simulink model "of_guidance"  (R2017b)
settings: Solver=FixedStepDiscrete  StartTime=0.0  StopTime=inf  FixedStep=0.01  RelTol=1e-3
undefined symbols (not defined in the file): Data, Data_SL_Info, DiscIntNeverNeededParam, Y_Velocity
libraries: robotlib x6, dspstat3 x5, simulink x3
settings Model: Creator=a  LastModifiedBy=a
settings OptimizationCC: PassReuseOutputArgsAs=Individual arguments  MaxStackSize=64
settings DebuggingCC: ParameterTunabilityLossMsg=error
settings HardwareCC: ProdBitPerPointer=32  ProdBitPerSizeT=32  ProdBitPerPtrDiffT=32  ProdLargestAtomicFloat=None  ProdIntDivRoundTo=Undefined  ProdEndianess=Unspecified  ProdWordSize=32  ProdHWDeviceType=Generic->Unspecified (assume 32-bit Generic)
settings SFSimCC: MATLABDynamicMemAlloc=off
settings RTWCC: SystemTargetFile=ert.tlc  HardwareBoard=Robot Operating System (ROS)  TemplateMakefile=ert_default_tmf  GenerateReport=on  Toolchain=Catkin  IncludeHyperlinkInReport=on  LaunchReport=on  TargetLang=C++  GenerateTraceInfo=on  GenerateTraceReport=on  GenerateTraceReportSl=on  GenerateTraceReportSf=on  GenerateTraceReportEml=on
settings CodeAppCC: ForceParamTrailComments=on  IgnoreCustomStorageClasses=off  OperatorAnnotations=on  SimulinkDataObjDesc=on  SFDataObjDesc=on  InsertBlockDesc=on

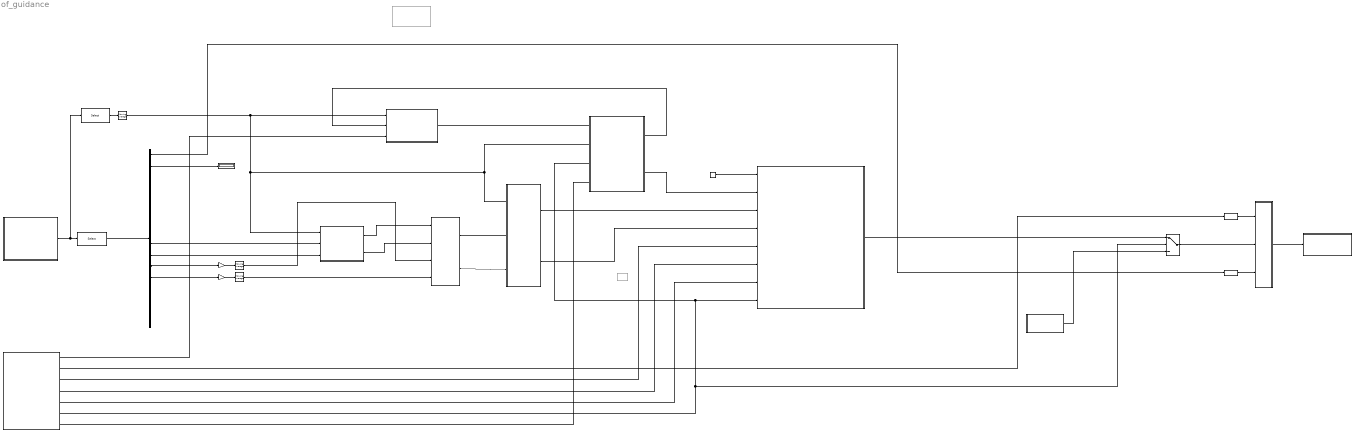
== system of_guidance ==
  Data Type Conversion3 : DataTypeConversion  OutDataTypeStr=single
  Data Type Conversion4 : DataTypeConversion  OutDataTypeStr=single
  Demux : Demux  Outputs=16
  P Moving Average : dspstat3/Moving Average  Method=Sliding window  SpecifyWindowLength=on  WindowLength=35  ForgettingFactor=0.9  SimulateUsing=Code generation
  Q Moving Average : dspstat3/Moving Average  Method=Sliding window  SpecifyWindowLength=on  WindowLength=35  ForgettingFactor=0.9  SimulateUsing=Code generation
  Selector : Selector  InputPortWidth=26  IndexOptions=Index vector (dialog)  Indices=[17:26 4 5 6 11 12 13]  OutputSizes=1
  Selector1 : Selector  InputPortWidth=26  IndexOptions=Index vector (dialog)  Indices=[7]  OutputSizes=1
  Sonar Moving Average : dspstat3/Moving Average  Method=Sliding window  SpecifyWindowLength=on  WindowLength=5  ForgettingFactor=0.9  SimulateUsing=Code generation
  Subsystem2 : Subsystem
  Subsystem5 : Subsystem
  Switch : Switch  Criteria=u2 > Threshold
  check_arm_status : Subsystem
  command_input : Subsystem
  command_output : Subsystem
  compensate_angular_velocity_effect_on_of : Subsystem
  "data_input " : Subsystem
  manual_control : Subsystem  mask{throttle=0.0, roll=0, pitch=0, yaw=0, mode=0}
  manual_throttle : Subsystem  Commented=on  mask{th=90}
  mode : Constant  Value=2
  p gain : Gain  Gain=3.1415 / 180.0
  pixel_per_sec_to_m_per_sec : Subsystem
  q gain : Gain  Gain=3.1415 / 180.0
  radio_command_frame_rate : Display
  throttle_handler_climb_mode : Subsystem
  velocity_control : Subsystem
  vy_setpoint1 : Constant  Commented=on  Value=Y_Velocity
  wires:
  command_input/5(vx_des) -> velocity_control/7(vx_setpoint)
  Selector/1 -> Demux/1
  pixel_per_sec_to_m_per_sec/2(vy(m/s)) -> compensate_angular_velocity_effect_on_of/2(vy)
  Demux/2 -> radio_command_frame_rate/1
  Switch/1 -> check_arm_status/2(command)
  command_input/6(take_off) -> Switch/2, velocity_control/8(Integrator_reset), throttle_handler_climb_mode/3(integrator_reset)
  Subsystem2/1(throttle_command) -> throttle_handler_climb_mode/1(desired_throttle)
  command_input/3(yaw_rate_des) -> velocity_control/5(yaw_des_rate)
  throttle_handler_climb_mode/1(z_controller_integrator_reset) -> Subsystem2/2(integrator_reset)
  command_input/1(z_des) -> Subsystem2/3(z_desired)
  command_input/4(vy_des) -> velocity_control/6(vy_setpoint)
  command_input/7(landing) -> throttle_handler_climb_mode/4(landing)
  Demux/12 -> q gain/1
  velocity_control/1(radio_command) -> Switch/1
  Subsystem5/2(vy_out) -> velocity_control/4(vy)
  Demux/11 -> p gain/1
  Demux/10 -> pixel_per_sec_to_m_per_sec/3(vy(pix/sec))
  "data_input "/1(data) -> Selector/1, Selector1/1
  command_input/2(arm_status) -> Data Type Conversion4/1
  Demux/9 -> pixel_per_sec_to_m_per_sec/2(vx(pix/sec))
  compensate_angular_velocity_effect_on_of/1(corrected_vx) -> Subsystem5/2(vx)
  p gain/1 -> P Moving Average/1
  q gain/1 -> Q Moving Average/1
  pixel_per_sec_to_m_per_sec/1(vx(m/s)) -> compensate_angular_velocity_effect_on_of/1(vx)
  P Moving Average/1 -> compensate_angular_velocity_effect_on_of/3(p)
  Data Type Conversion4/1 -> check_arm_status/1(arm)
  manual_control/1(commands) -> Switch/3
  Subsystem5/1(vx_out) -> velocity_control/3(vx)
  Data Type Conversion3/1 -> check_arm_status/3(motors_on)
  check_arm_status/1(Out) -> command_output/1(command)
  Sonar Moving Average/1 -> pixel_per_sec_to_m_per_sec/1(height), Subsystem5/1(height), throttle_handler_climb_mode/2(height), Subsystem2/1(measured_height)
  mode/1 -> velocity_control/1(mode)
  throttle_handler_climb_mode/2(throttle) -> velocity_control/2(throttle)
  Demux/1 -> Data Type Conversion3/1
  Selector1/1 -> Sonar Moving Average/1
  compensate_angular_velocity_effect_on_of/2(corrected_vy) -> Subsystem5/3(vy)
  Q Moving Average/1 -> compensate_angular_velocity_effect_on_of/4(q)

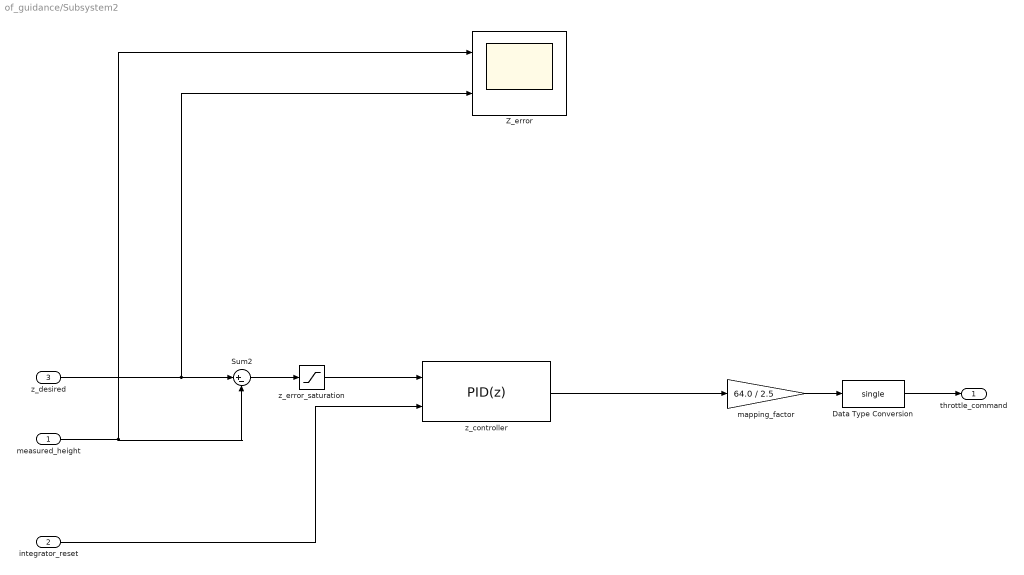
== system of_guidance/Subsystem2 ==
  measured_height : Inport
  integrator_reset : Inport  Port=2
  z_desired : Inport  Port=3
  Data Type Conversion : DataTypeConversion  OutDataTypeStr=single
  Sum2 : Sum  Inputs=|+-
  Z_error : Scope  NumInputPorts=2
  mapping_factor : Gain  Gain=64.0 / 2.5
  z_controller : simulink/Continuous/PID Controller  Controller=PID  TimeDomain=Discrete-time  SampleTime=-1  IntegratorMethod=Forward Euler  FilterMethod=Forward Euler  Form=Parallel  UseFilter=on  ControllerParametersSource=internal  P=1.5  I=0.3  D=0.2  N=100  InitialConditionSource=internal  InitialConditionForIntegrator=0  InitialConditionForFilter=0  ExternalReset=rising  LimitOutput=on  UpperSaturationLimit=1.0  LowerSaturationLimit=-1.0  LinearizeAsGain=off  AntiWindupMode=none  Kb=1  TrackingMode=off  Kt=1  PParamMin=[]  PParamMax=[]  IParamMin=[]  IParamMax=[]  DParamMin=[]  DParamMax=[]  NParamMin=[]  NParamMax=[]  KbParamMin=[]  KbParamMax=[]  KtParamMin=[]  KtParamMax=[]  POutMin=[]  POutMax=[]  IOutMin=[]  IOutMax=[]  DOutMin=[]  DOutMax=[]  NOutMin=[]  NOutMax=[]  KbOutMin=[]  KbOutMax=[]  KtOutMin=[]  KtOutMax=[]  IntegratorOutMin=[]  IntegratorOutMax=[]  FilterOutMin=[]  FilterOutMax=[]  SumOutMin=[]  SumOutMax=[]  SumI1OutMin=[]  SumI1OutMax=[]  SumI2OutMin=[]  SumI2OutMax=[]  SumI3OutMin=[]  SumI3OutMax=[]  SumDOutMin=[]  SumDOutMax=[]  SaturationOutMin=[]  SaturationOutMax=[]  IntegratorContinuousStateAttributes=''  IntegratorStateMustResolveToSignalObject=off  IntegratorRTWStateStorageClass=Auto  FilterContinuousStateAttributes=''  FilterStateMustResolveToSignalObject=off  FilterRTWStateStorageClass=Auto  DifferentiatorICPrevScaledInput=0  DifferentiatorOutMin=[]  DifferentiatorOutMax=[]  InitialConditionSetting=State (most efficient)  FilterDiffOutCoefMin=[]  FilterDiffOutCoefMax=[]  SumDenOutMin=[]  SumDenOutMax=[]  SumNumOutMin=[]  SumNumOutMax=[]  ReciprocalOutMin=[]  ReciprocalOutMax=[]  DivideOutMin=[]  DivideOutMax=[]  TunerSelectOption=Transfer Function Based (PID Tuner App)
  z_error_saturation : Saturate  UpperLimit=1  LowerLimit=-1
  throttle_command : Outport
  wires:
  integrator_reset/1 -> z_controller/2
  mapping_factor/1 -> Data Type Conversion/1
  measured_height/1 -> Sum2/2, Z_error/1
  z_desired/1 -> Z_error/2, Sum2/1
  Sum2/1 -> z_error_saturation/1
  z_error_saturation/1 -> z_controller/1
  z_controller/1 -> mapping_factor/1
  Data Type Conversion/1 -> throttle_command/1

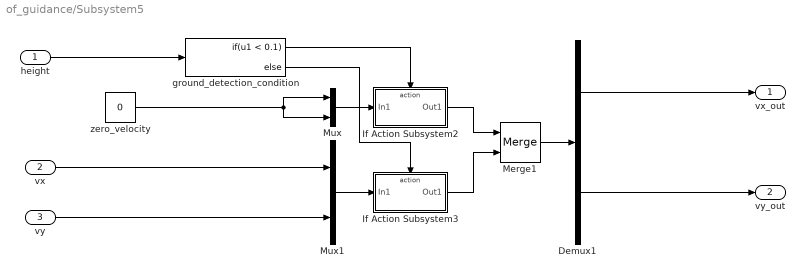
== system of_guidance/Subsystem5 ==
  height : Inport
  vx : Inport  Port=2
  vy : Inport  Port=3
  Demux1 : Demux  Outputs=2
  If Action Subsystem2 : Subsystem  TreatAsAtomicUnit=on
  If Action Subsystem3 : Subsystem  TreatAsAtomicUnit=on
  Merge1 : Merge
  Mux : Mux  Inputs=2
  Mux1 : Mux  Inputs=2
  ground_detection_condition : If  IfExpression=u1 < 0.1
  zero_velocity : Constant  Value=0
  vx_out : Outport
  vy_out : Outport  Port=2
  wires:
  vy/1 -> Mux1/2
  vx/1 -> Mux1/1
  height/1 -> ground_detection_condition/1
  Demux1/1 -> vx_out/1
  zero_velocity/1 -> Mux/2, Mux/1
  Demux1/2 -> vy_out/1
  ground_detection_condition/1 -> If Action Subsystem2/Action
  If Action Subsystem3/1(Out1) -> Merge1/2
  Merge1/1 -> Demux1/1
  Mux1/1 -> If Action Subsystem3/1(In1)
  ground_detection_condition/2 -> If Action Subsystem3/Action
  If Action Subsystem2/1(Out1) -> Merge1/1
  Mux/1 -> If Action Subsystem2/1(In1)

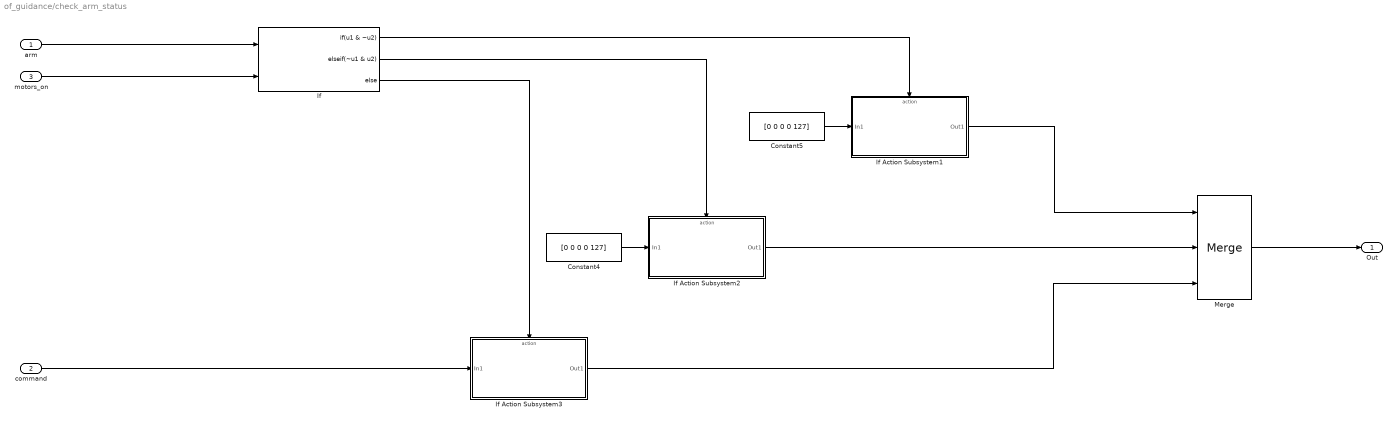
== system of_guidance/check_arm_status ==
  arm : Inport
  command : Inport  Port=2
  motors_on : Inport  Port=3
  Constant4 : Constant  Value=[0 0 0 0 127]
  Constant5 : Constant  Value=[0 0 0 0 127]
  If : If  NumInputs=2  IfExpression=u1 & ~u2  ElseIfExpressions=~u1 & u2
  If Action Subsystem1 : Subsystem  TreatAsAtomicUnit=on
  If Action Subsystem2 : Subsystem  TreatAsAtomicUnit=on
  If Action Subsystem3 : Subsystem  TreatAsAtomicUnit=on
  Merge : Merge  Inputs=3
  Out : Outport
  wires:
  If/1 -> If Action Subsystem1/Action
  Constant4/1 -> If Action Subsystem2/1(In1)
  If/3 -> If Action Subsystem3/Action
  Constant5/1 -> If Action Subsystem1/1(In1)
  If/2 -> If Action Subsystem2/Action
  If Action Subsystem2/1(Out1) -> Merge/2
  motors_on/1 -> If/2
  command/1 -> If Action Subsystem3/1(In1)
  If Action Subsystem1/1(Out1) -> Merge/1
  If Action Subsystem3/1(Out1) -> Merge/3
  arm/1 -> If/1
  Merge/1 -> Out/1

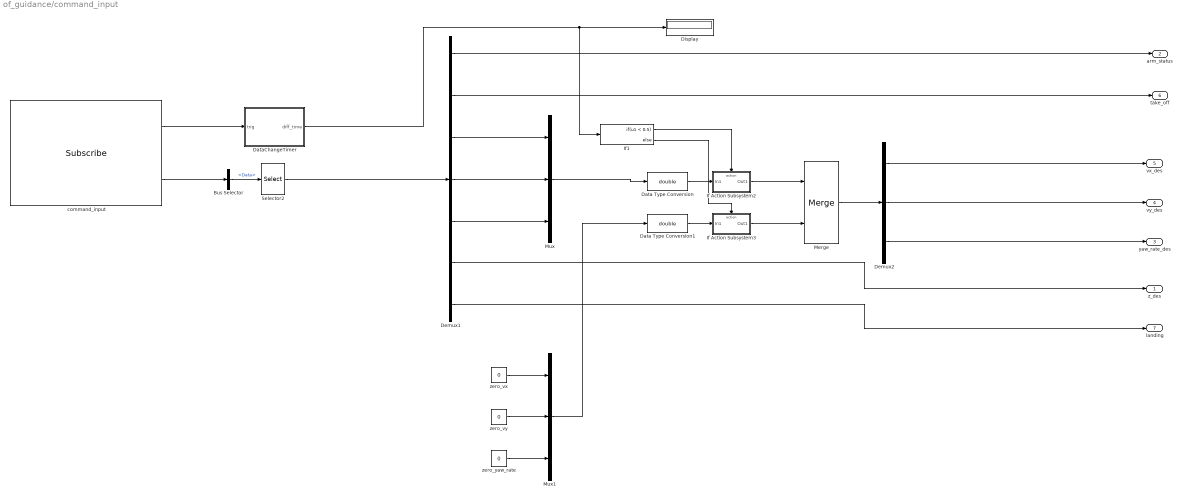
== system of_guidance/command_input ==
  Bus Selector : BusSelector  OutputSignals=Data
  Data Type Conversion : DataTypeConversion  OutDataTypeStr=double
  Data Type Conversion1 : DataTypeConversion  OutDataTypeStr=double
  DataChangeTimer : Subsystem
  Demux1 : Demux  Outputs=7
  Demux2 : Demux  Outputs=3
  Display : Display
  If Action Subsystem2 : Subsystem  TreatAsAtomicUnit=on
  If Action Subsystem3 : Subsystem  TreatAsAtomicUnit=on
  If1 : If  IfExpression=u1 < 0.5
  Merge : Merge
  Mux : Mux  Inputs=3
  Mux1 : Mux  Inputs=3
  Selector2 : Selector  InputPortWidth=128  IndexOptions=Index vector (dialog)  Indices=[1 2 3 4 5 6 7]  OutputSizes=1
  command_input : robotlib/Subscribe  SourceLibraryInfo=This block requires Robotics System Toolbox  topicSource=Specify your own  topic=/quadrotor_1/road_following_cmd  messageType=std_msgs/Float32MultiArray  sampleTime=-1  messageQueueLength=1
      settings: SourceProductBaseCode=RO
  zero_vx : Constant  Value=0
  zero_vy : Constant  Value=0
  zero_yaw_rate : Constant  Value=0
  z_des : Outport
  arm_status : Outport  Port=2
  yaw_rate_des : Outport  Port=3
  vy_des : Outport  Port=4
  vx_des : Outport  Port=5
  take_off : Outport  Port=6
  landing : Outport  Port=7
  wires:
  DataChangeTimer/1(diff_time) -> If1/1, Display/1
  If1/2 -> If Action Subsystem3/Action
  Demux1/5 -> Mux/3
  Demux1/1 -> arm_status/1
  Demux2/1 -> vx_des/1
  If1/1 -> If Action Subsystem2/Action
  Demux1/4 -> Mux/2
  command_input/1 -> DataChangeTimer/1(trig)
  Mux/1 -> Data Type Conversion/1
  command_input/2 -> Bus Selector/1
  Bus Selector/1 -> Selector2/1  "<Data>"
  Demux1/2 -> take_off/1
  Demux2/2 -> vy_des/1
  Demux1/6 -> z_des/1
  Demux2/3 -> yaw_rate_des/1
  Selector2/1 -> Demux1/1
  zero_yaw_rate/1 -> Mux1/3
  zero_vx/1 -> Mux1/1
  Mux1/1 -> Data Type Conversion1/1
  zero_vy/1 -> Mux1/2
  Demux1/3 -> Mux/1
  Merge/1 -> Demux2/1
  Demux1/7 -> landing/1
  If Action Subsystem2/1(Out1) -> Merge/1
  If Action Subsystem3/1(Out1) -> Merge/2
  Data Type Conversion/1 -> If Action Subsystem2/1(In1)
  Data Type Conversion1/1 -> If Action Subsystem3/1(In1)

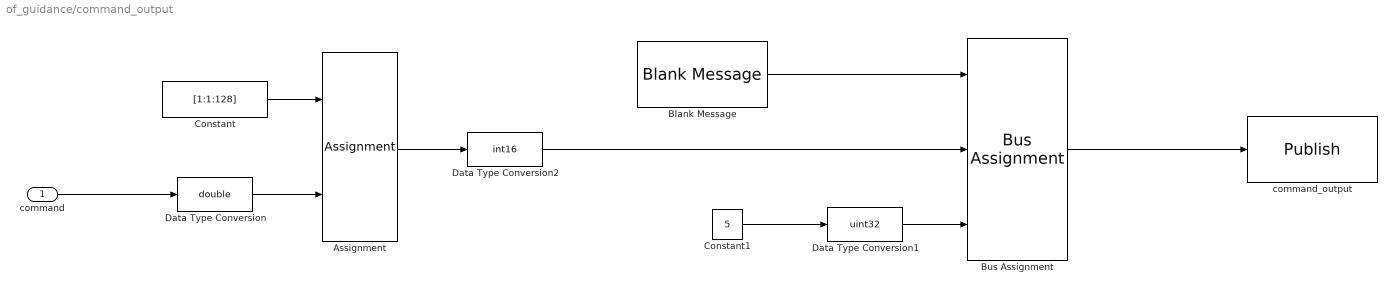
== system of_guidance/command_output ==
  command : Inport
  Assignment : Assignment  DiagnosticForDimensions=Warning  IndexOptions=Index vector (dialog)  Indices=[1 2 3 4 5]  OutputSizes=1
  Blank Message : robotlib/Blank Message  SourceLibraryInfo=This block requires Robotics System Toolbox  messageType=std_msgs/Int16MultiArray  SampleTime=inf
      settings: SourceProductBaseCode=RO
  Bus Assignment : BusAssignment  AssignedSignals=Data,Data_SL_Info.CurrentLength
  Constant : Constant  Value=[1:1:128]
  Constant1 : Constant  Value=5
  Data Type Conversion : DataTypeConversion  OutDataTypeStr=double
  Data Type Conversion1 : DataTypeConversion  OutDataTypeStr=uint32
  Data Type Conversion2 : DataTypeConversion  OutDataTypeStr=int16
  "command_output " : robotlib/Publish  SourceLibraryInfo=This block requires Robotics System Toolbox  topicSource=Select from ROS network  topic=/quadrotor_1/rpyt_command  messageType=std_msgs/Int16MultiArray  messageQueueLength=1
      settings: SourceProductBaseCode=RO
  wires:
  Constant1/1 -> Data Type Conversion1/1
  Data Type Conversion1/1 -> Bus Assignment/3
  Bus Assignment/1 -> "command_output "/1
  Data Type Conversion2/1 -> Bus Assignment/2
  Assignment/1 -> Data Type Conversion2/1
  Blank Message/1 -> Bus Assignment/1
  Data Type Conversion/1 -> Assignment/2
  command/1 -> Data Type Conversion/1
  Constant/1 -> Assignment/1

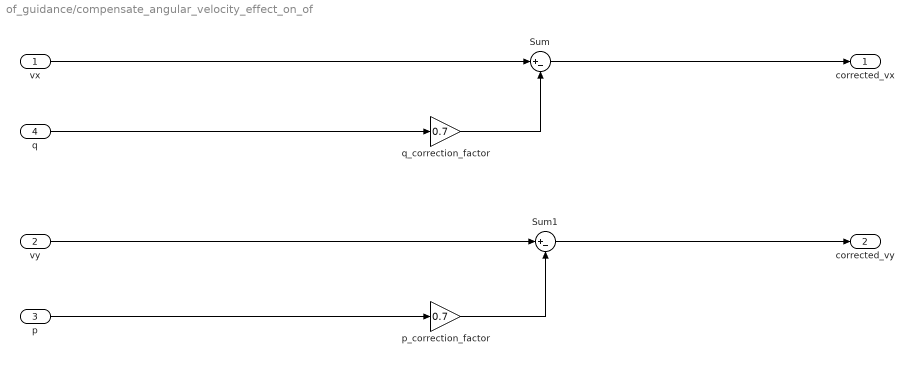
== system of_guidance/compensate_angular_velocity_effect_on_of ==
  vx : Inport
  vy : Inport  Port=2
  p : Inport  Port=3
  q : Inport  Port=4
  Sum : Sum  Inputs=|+-
  Sum1 : Sum  Inputs=|+-
  p_correction_factor : Gain  Gain=0.7
  q_correction_factor : Gain  Gain=0.7
  corrected_vx : Outport
  corrected_vy : Outport  Port=2
  wires:
  vx/1 -> Sum/1
  vy/1 -> Sum1/1
  q/1 -> q_correction_factor/1
  p/1 -> p_correction_factor/1
  Sum1/1 -> corrected_vy/1
  Sum/1 -> corrected_vx/1
  p_correction_factor/1 -> Sum1/2
  q_correction_factor/1 -> Sum/2

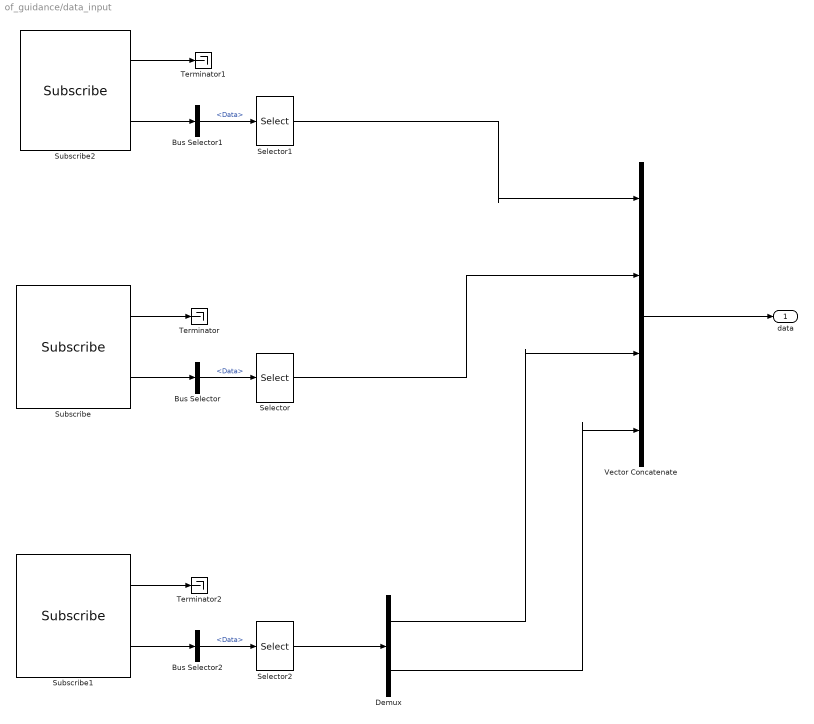
== system of_guidance/data_input  ==
  Bus Selector : BusSelector  OutputSignals=Data
  Bus Selector1 : BusSelector  OutputSignals=Data
  Bus Selector2 : BusSelector  OutputSignals=Data
  Demux : Demux  Outputs=2
  Selector : Selector  InputPortWidth=128  IndexOptions=Index vector (dialog)  Indices=[1 2 3 4 5 6]  OutputSizes=1
  Selector1 : Selector  InputPortWidth=128  IndexOptions=Index vector (dialog)  Indices=[1 2 3 4 5 6 7 8 9 10 11 12 13 14 15 16 17 18]  OutputSizes=1
  Selector2 : Selector  InputPortWidth=128  IndexOptions=Index vector (dialog)  Indices=[1 2]  OutputSizes=1
  Subscribe : robotlib/Subscribe  SourceLibraryInfo=This block requires Robotics System Toolbox  topicSource=Select from ROS network  topic=/quadrotor_1/nav  messageType=std_msgs/Float32MultiArray  sampleTime=-1  messageQueueLength=1
      settings: SourceProductBaseCode=RO
  Subscribe1 : robotlib/Subscribe  SourceLibraryInfo=This block requires Robotics System Toolbox  topicSource=Select from ROS network  topic=/quadrotor_1/optical_flow  messageType=std_msgs/Float32MultiArray  sampleTime=-1  messageQueueLength=1
      settings: SourceProductBaseCode=RO
  Subscribe2 : robotlib/Subscribe  SourceLibraryInfo=This block requires Robotics System Toolbox  topicSource=Select from ROS network  topic=/quadrotor_1/sensor_data  messageType=std_msgs/Float32MultiArray  sampleTime=-1  messageQueueLength=1
      settings: SourceProductBaseCode=RO
  Terminator : Terminator
  Terminator1 : Terminator
  Terminator2 : Terminator
  Vector Concatenate : Concatenate  NumInputs=4
  data : Outport
  wires:
  Subscribe/1 -> Terminator/1
  Selector/1 -> Vector Concatenate/2
  Subscribe2/1 -> Terminator1/1
  Subscribe2/2 -> Bus Selector1/1
  Subscribe/2 -> Bus Selector/1
  Bus Selector/1 -> Selector/1  "<Data>"
  Bus Selector1/1 -> Selector1/1  "<Data>"
  Selector1/1 -> Vector Concatenate/1
  Vector Concatenate/1 -> data/1
  Subscribe1/2 -> Bus Selector2/1
  Subscribe1/1 -> Terminator2/1
  Bus Selector2/1 -> Selector2/1  "<Data>"
  Selector2/1 -> Demux/1
  Demux/1 -> Vector Concatenate/3
  Demux/2 -> Vector Concatenate/4

== system of_guidance/manual_control ==
  Constant : Constant  Value=[mode throttle roll pitch yaw]
  commands : Outport
  wires:
  Constant/1 -> commands/1

== system of_guidance/manual_throttle ==
  mode1 : Constant  Value=th
  Out1 : Outport
  wires:
  mode1/1 -> Out1/1

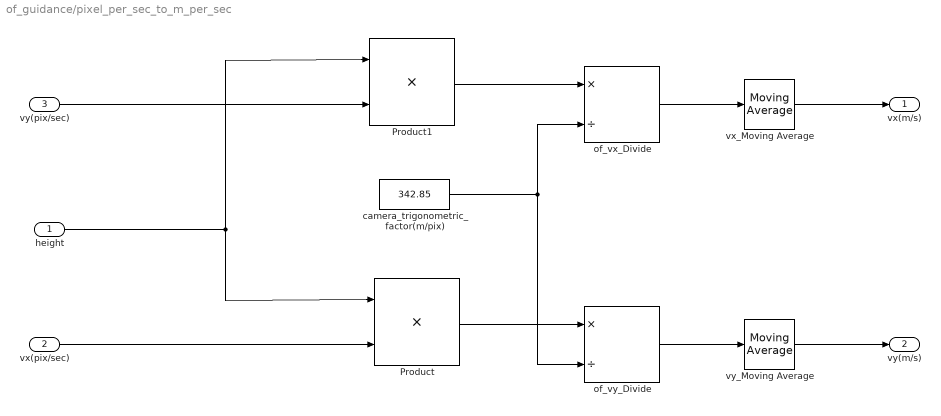
== system of_guidance/pixel_per_sec_to_m_per_sec ==
  height : Inport
  vx(pix/sec) : Inport  Port=2
  vy(pix/sec) : Inport  Port=3
  Product : Product
  Product1 : Product
  camera_trigonometric_factor(m/pix) : Constant  Value=342.85
  of_vx_Divide : Product  Inputs=*/
  of_vy_Divide : Product  Inputs=*/
  vx_Moving Average : dspstat3/Moving Average  Method=Sliding window  SpecifyWindowLength=on  WindowLength=35  ForgettingFactor=0.9  SimulateUsing=Code generation
  vy_Moving Average : dspstat3/Moving Average  Method=Sliding window  SpecifyWindowLength=on  WindowLength=35  ForgettingFactor=0.9  SimulateUsing=Code generation
  vx(m/s) : Outport
  vy(m/s) : Outport  Port=2
  wires:
  height/1 -> Product1/1, Product/1
  of_vx_Divide/1 -> vx_Moving Average/1
  Product/1 -> of_vy_Divide/1
  Product1/1 -> of_vx_Divide/1
  vy_Moving Average/1 -> vy(m/s)/1
  vx_Moving Average/1 -> vx(m/s)/1
  of_vy_Divide/1 -> vy_Moving Average/1
  vy(pix/sec)/1 -> Product1/2
  camera_trigonometric_factor(m/pix)/1 -> of_vy_Divide/2, of_vx_Divide/2
  vx(pix/sec)/1 -> Product/2

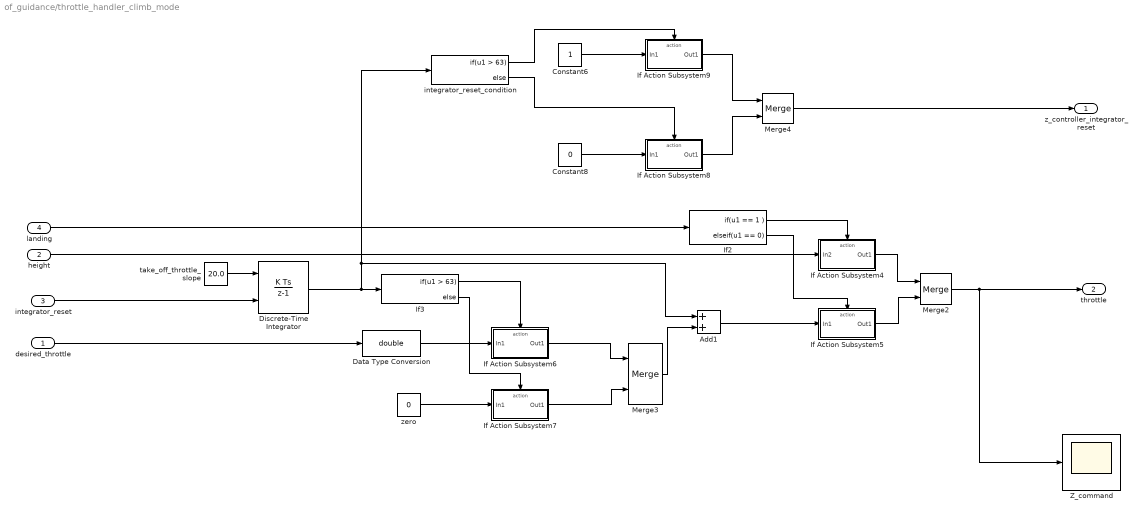
== system of_guidance/throttle_handler_climb_mode ==
  desired_throttle : Inport
  height : Inport  Port=2
  integrator_reset : Inport  Port=3
  landing : Inport  Port=4
  Add1 : Sum
  Constant6 : Constant
  Constant8 : Constant  Value=0
  Data Type Conversion : DataTypeConversion  OutDataTypeStr=double
  Discrete-Time Integrator : DiscreteIntegrator  ExternalReset=either  InitialConditionSetting=State (most efficient)  SampleTime=-1  LimitOutput=on  UpperSaturationLimit=64  LowerSaturationLimit=0  ICPrevOutput=DiscIntNeverNeededParam  ICPrevScaledInput=DiscIntNeverNeededParam
  If Action Subsystem4 : Subsystem  TreatAsAtomicUnit=on
  If Action Subsystem5 : Subsystem  TreatAsAtomicUnit=on
  If Action Subsystem6 : Subsystem  TreatAsAtomicUnit=on
  If Action Subsystem7 : Subsystem  TreatAsAtomicUnit=on
  If Action Subsystem8 : Subsystem  TreatAsAtomicUnit=on
  If Action Subsystem9 : Subsystem  TreatAsAtomicUnit=on
  If2 : If  IfExpression=u1 == 1  ElseIfExpressions=u1 == 0  ShowElse=off
  If3 : If  IfExpression=u1 > 63
  Merge2 : Merge
  Merge3 : Merge
  Merge4 : Merge
  Z_command : Scope
  integrator_reset_condition : If  IfExpression=u1 > 63
  take_off_throttle_slope : Constant  Value=20.0
  zero : Constant  Value=0
  z_controller_integrator_reset : Outport
  throttle : Outport  Port=2
  wires:
  height/1 -> If Action Subsystem4/1(In2)
  integrator_reset/1 -> Discrete-Time Integrator/2
  If3/2 -> If Action Subsystem7/Action
  If Action Subsystem5/1(Out1) -> Merge2/2
  If Action Subsystem4/1(Out1) -> Merge2/1
  zero/1 -> If Action Subsystem7/1(In1)
  If Action Subsystem7/1(Out1) -> Merge3/2
  Merge3/1 -> Add1/2
  Discrete-Time Integrator/1 -> integrator_reset_condition/1, Add1/1, If3/1
  landing/1 -> If2/1
  Add1/1 -> If Action Subsystem5/1(In1)
  Merge2/1 -> Z_command/1, throttle/1
  If3/1 -> If Action Subsystem6/Action
  desired_throttle/1 -> Data Type Conversion/1
  If2/1 -> If Action Subsystem4/Action
  If2/2 -> If Action Subsystem5/Action
  take_off_throttle_slope/1 -> Discrete-Time Integrator/1
  integrator_reset_condition/1 -> If Action Subsystem9/Action
  Merge4/1 -> z_controller_integrator_reset/1
  integrator_reset_condition/2 -> If Action Subsystem8/Action
  If Action Subsystem8/1(Out1) -> Merge4/2
  If Action Subsystem9/1(Out1) -> Merge4/1
  Constant8/1 -> If Action Subsystem8/1(In1)
  Constant6/1 -> If Action Subsystem9/1(In1)
  If Action Subsystem6/1(Out1) -> Merge3/1
  Data Type Conversion/1 -> If Action Subsystem6/1(In1)

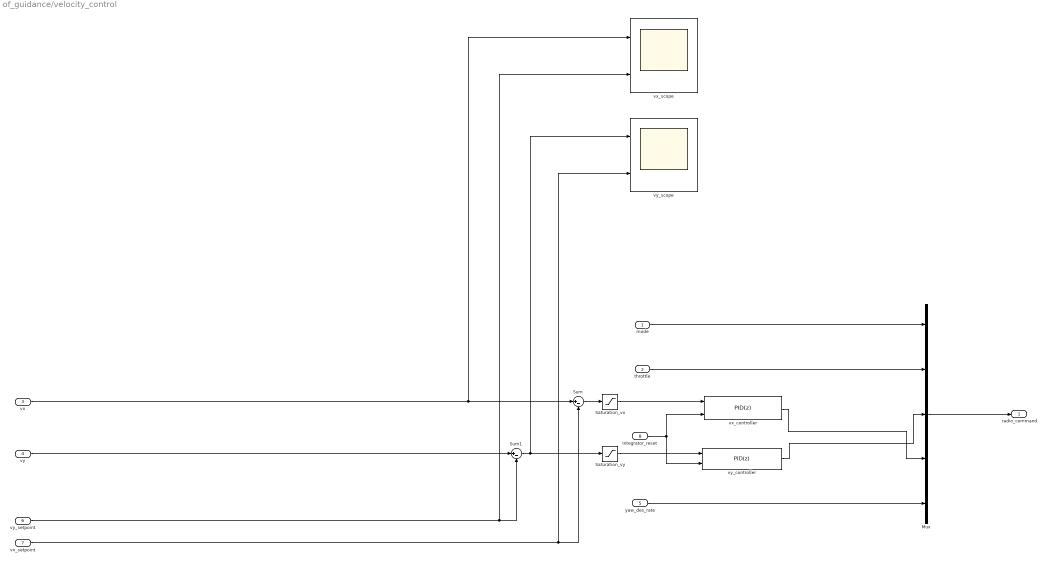
== system of_guidance/velocity_control ==
  mode : Inport
  throttle : Inport  Port=2
  vx : Inport  Port=3
  vy : Inport  Port=4
  yaw_des_rate : Inport  Port=5
  vy_setpoint : Inport  Port=6
  vx_setpoint : Inport  Port=7
  Integrator_reset : Inport  Port=8
  Mux : Mux  Inputs=5
  Saturation_vx : Saturate  UpperLimit=1  LowerLimit=-1
  Saturation_vy : Saturate  UpperLimit=1  LowerLimit=-1
  Sum : Sum  Inputs=|+-
  Sum1 : Sum  Inputs=|+-
  vx_controller : simulink/Continuous/PID Controller  Controller=PID  TimeDomain=Discrete-time  SampleTime=-1  IntegratorMethod=Forward Euler  FilterMethod=Forward Euler  Form=Parallel  UseFilter=on  ControllerParametersSource=internal  P=20  I=20  D=0  N=100  InitialConditionSource=internal  InitialConditionForIntegrator=0  InitialConditionForFilter=0  ExternalReset=either  LimitOutput=on  UpperSaturationLimit=127  LowerSaturationLimit=-127  LinearizeAsGain=off  AntiWindupMode=none  Kb=1  TrackingMode=off  Kt=1  PParamMin=[]  PParamMax=[]  IParamMin=[]  IParamMax=[]  DParamMin=[]  DParamMax=[]  NParamMin=[]  NParamMax=[]  KbParamMin=[]  KbParamMax=[]  KtParamMin=[]  KtParamMax=[]  POutMin=[]  POutMax=[]  IOutMin=[]  IOutMax=[]  DOutMin=[]  DOutMax=[]  NOutMin=[]  NOutMax=[]  KbOutMin=[]  KbOutMax=[]  KtOutMin=[]  KtOutMax=[]  IntegratorOutMin=[]  IntegratorOutMax=[]  FilterOutMin=[]  FilterOutMax=[]  SumOutMin=[]  SumOutMax=[]  SumI1OutMin=[]  SumI1OutMax=[]  SumI2OutMin=[]  SumI2OutMax=[]  SumI3OutMin=[]  SumI3OutMax=[]  SumDOutMin=[]  SumDOutMax=[]  SaturationOutMin=[]  SaturationOutMax=[]  IntegratorContinuousStateAttributes=''  IntegratorStateMustResolveToSignalObject=off  IntegratorRTWStateStorageClass=Auto  FilterContinuousStateAttributes=''  FilterStateMustResolveToSignalObject=off  FilterRTWStateStorageClass=Auto  DifferentiatorICPrevScaledInput=0  DifferentiatorOutMin=[]  DifferentiatorOutMax=[]  InitialConditionSetting=State (most efficient)  FilterDiffOutCoefMin=[]  FilterDiffOutCoefMax=[]  SumDenOutMin=[]  SumDenOutMax=[]  SumNumOutMin=[]  SumNumOutMax=[]  ReciprocalOutMin=[]  ReciprocalOutMax=[]  DivideOutMin=[]  DivideOutMax=[]  TunerSelectOption=Transfer Function Based (PID Tuner App)
  vx_scope : Scope  NumInputPorts=2
  vy_controller : simulink/Continuous/PID Controller  Controller=PID  TimeDomain=Discrete-time  SampleTime=-1  IntegratorMethod=Forward Euler  FilterMethod=Forward Euler  Form=Parallel  UseFilter=on  ControllerParametersSource=internal  P=20  I=20  D=0  N=100  InitialConditionSource=internal  InitialConditionForIntegrator=0  InitialConditionForFilter=0  ExternalReset=either  LimitOutput=on  UpperSaturationLimit=127  LowerSaturationLimit=-127  LinearizeAsGain=off  AntiWindupMode=none  Kb=1  TrackingMode=off  Kt=1  PParamMin=[]  PParamMax=[]  IParamMin=[]  IParamMax=[]  DParamMin=[]  DParamMax=[]  NParamMin=[]  NParamMax=[]  KbParamMin=[]  KbParamMax=[]  KtParamMin=[]  KtParamMax=[]  POutMin=[]  POutMax=[]  IOutMin=[]  IOutMax=[]  DOutMin=[]  DOutMax=[]  NOutMin=[]  NOutMax=[]  KbOutMin=[]  KbOutMax=[]  KtOutMin=[]  KtOutMax=[]  IntegratorOutMin=[]  IntegratorOutMax=[]  FilterOutMin=[]  FilterOutMax=[]  SumOutMin=[]  SumOutMax=[]  SumI1OutMin=[]  SumI1OutMax=[]  SumI2OutMin=[]  SumI2OutMax=[]  SumI3OutMin=[]  SumI3OutMax=[]  SumDOutMin=[]  SumDOutMax=[]  SaturationOutMin=[]  SaturationOutMax=[]  IntegratorContinuousStateAttributes=''  IntegratorStateMustResolveToSignalObject=off  IntegratorRTWStateStorageClass=Auto  FilterContinuousStateAttributes=''  FilterStateMustResolveToSignalObject=off  FilterRTWStateStorageClass=Auto  DifferentiatorICPrevScaledInput=0  DifferentiatorOutMin=[]  DifferentiatorOutMax=[]  InitialConditionSetting=State (most efficient)  FilterDiffOutCoefMin=[]  FilterDiffOutCoefMax=[]  SumDenOutMin=[]  SumDenOutMax=[]  SumNumOutMin=[]  SumNumOutMax=[]  ReciprocalOutMin=[]  ReciprocalOutMax=[]  DivideOutMin=[]  DivideOutMax=[]  TunerSelectOption=Transfer Function Based (PID Tuner App)
  vy_scope : Scope  NumInputPorts=2
  radio_command : Outport
  wires:
  vy/1 -> Sum1/1
  vy_setpoint/1 -> vx_scope/2, Sum1/2
  Sum1/1 -> Saturation_vy/1, vy_scope/1
  vy_controller/1 -> Mux/3
  Mux/1 -> radio_command/1
  vx/1 -> vx_scope/1, Sum/1
  Sum/1 -> Saturation_vx/1
  vx_setpoint/1 -> vy_scope/2, Sum/2
  mode/1 -> Mux/1
  yaw_des_rate/1 -> Mux/5
  throttle/1 -> Mux/2
  vx_controller/1 -> Mux/4
  Integrator_reset/1 -> vy_controller/2, vx_controller/2
  Saturation_vx/1 -> vx_controller/1
  Saturation_vy/1 -> vy_controller/1

== system of_guidance/Subsystem5/If Action Subsystem2 ==
  In1 : Inport
  Action Port : ActionPort
  Out1 : Outport
  wires:
  In1/1 -> Out1/1

== system of_guidance/Subsystem5/If Action Subsystem3 ==
  In1 : Inport
  Action Port : ActionPort
  Out1 : Outport
  wires:
  In1/1 -> Out1/1

== system of_guidance/check_arm_status/If Action Subsystem1 ==
  In1 : Inport
  Action Port : ActionPort
  Out1 : Outport
  wires:
  In1/1 -> Out1/1

== system of_guidance/check_arm_status/If Action Subsystem2 ==
  In1 : Inport
  Action Port : ActionPort
  Out1 : Outport
  wires:
  In1/1 -> Out1/1

== system of_guidance/check_arm_status/If Action Subsystem3 ==
  In1 : Inport
  Action Port : ActionPort
  Out1 : Outport
  wires:
  In1/1 -> Out1/1

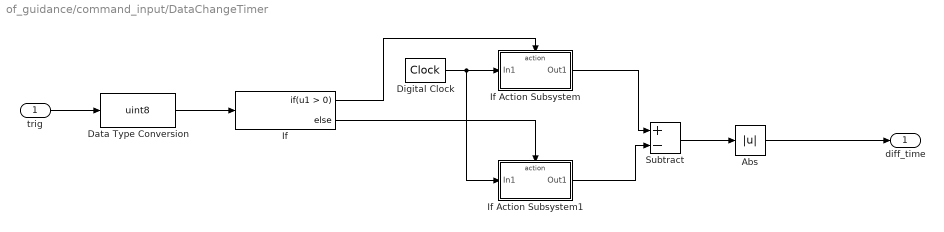
== system of_guidance/command_input/DataChangeTimer ==
  trig : Inport
  Abs : Abs
  Data Type Conversion : DataTypeConversion  OutDataTypeStr=uint8
  Digital Clock : DigitalClock  SampleTime=0.01
  If : If
  If Action Subsystem : Subsystem  TreatAsAtomicUnit=on
  If Action Subsystem1 : Subsystem  TreatAsAtomicUnit=on
  Subtract : Sum  Inputs=+-
  diff_time : Outport
  wires:
  If Action Subsystem1/1(Out1) -> Subtract/2
  Subtract/1 -> Abs/1
  trig/1 -> Data Type Conversion/1
  Abs/1 -> diff_time/1
  If Action Subsystem/1(Out1) -> Subtract/1
  Digital Clock/1 -> If Action Subsystem1/1(In1), If Action Subsystem/1(In1)
  If/2 -> If Action Subsystem1/Action
  If/1 -> If Action Subsystem/Action
  Data Type Conversion/1 -> If/1

== system of_guidance/command_input/If Action Subsystem2 ==
  In1 : Inport
  Action Port : ActionPort
  Out1 : Outport
  wires:
  In1/1 -> Out1/1

== system of_guidance/command_input/If Action Subsystem3 ==
  In1 : Inport
  Action Port : ActionPort
  Out1 : Outport
  wires:
  In1/1 -> Out1/1

== system of_guidance/throttle_handler_climb_mode/If Action Subsystem4 ==
  In2 : Inport
  Action Port : ActionPort
  Constant1 : Constant  Value=0
  Constant4 : Constant  Value=44
  If : If  IfExpression=u1 < 0.1
  If Action Subsystem : Subsystem  TreatAsAtomicUnit=on
  If Action Subsystem1 : Subsystem  TreatAsAtomicUnit=on
  Merge : Merge
  Out1 : Outport
  wires:
  Merge/1 -> Out1/1
  If/1 -> If Action Subsystem/Action
  If/2 -> If Action Subsystem1/Action
  Constant1/1 -> If Action Subsystem/1(In1)
  In2/1 -> If/1
  Constant4/1 -> If Action Subsystem1/1(In1)
  If Action Subsystem/1(Out1) -> Merge/1
  If Action Subsystem1/1(Out1) -> Merge/2

== system of_guidance/throttle_handler_climb_mode/If Action Subsystem5 ==
  In1 : Inport
  Action Port : ActionPort
  Out1 : Outport
  wires:
  In1/1 -> Out1/1

== system of_guidance/throttle_handler_climb_mode/If Action Subsystem6 ==
  In1 : Inport
  Action Port : ActionPort
  Out1 : Outport
  wires:
  In1/1 -> Out1/1

== system of_guidance/throttle_handler_climb_mode/If Action Subsystem7 ==
  In1 : Inport
  Action Port : ActionPort
  Out1 : Outport
  wires:
  In1/1 -> Out1/1

== system of_guidance/throttle_handler_climb_mode/If Action Subsystem8 ==
  In1 : Inport
  Action Port : ActionPort
  Out1 : Outport
  wires:
  In1/1 -> Out1/1

== system of_guidance/throttle_handler_climb_mode/If Action Subsystem9 ==
  In1 : Inport
  Action Port : ActionPort
  Out1 : Outport
  wires:
  In1/1 -> Out1/1

== system of_guidance/command_input/DataChangeTimer/If Action Subsystem ==
  In1 : Inport
  Action Port : ActionPort
  Out1 : Outport
  wires:
  In1/1 -> Out1/1

== system of_guidance/command_input/DataChangeTimer/If Action Subsystem1 ==
  In1 : Inport
  Action Port : ActionPort
  Out1 : Outport
  wires:
  In1/1 -> Out1/1

== system of_guidance/throttle_handler_climb_mode/If Action Subsystem4/If Action Subsystem ==
  In1 : Inport
  Action Port : ActionPort
  Out1 : Outport
  wires:
  In1/1 -> Out1/1

== system of_guidance/throttle_handler_climb_mode/If Action Subsystem4/If Action Subsystem1 ==
  In1 : Inport
  Action Port : ActionPort
  Out1 : Outport
  wires:
  In1/1 -> Out1/1
